simulink model "hiv_model_ekf"  (R2020b)
settings: Solver=VariableStepAuto  StartTime=0.0  StopTime=10.0  RelTol=1e-3
values from neighbouring files (symbols this model uses):
  Delta = 0.01    [init.m]
  P_0 = [diag((Theta*0.3).^2),zeros(6,3);zeros(3,9)]    [init.m]
  Theta = block.DialogPrm(2).Data    [hiv_model.m]    (also in init.m = [0.25 50 0.25 10 0.01 0.0045]')
  W_k = zeros(9,9)    [init.m]
  xdash0 = [1000 550 0.0001]'    [init.m]
  xdash12RL = block.DialogPrm(3).Data    [hiv_model.m]    (also in init.m = [1000 550]')
  Z_k = zeros(3,3);Z_k(1,1)=100;Z_k(2,2)=100;Z_k(3,3)=1e-5    [init.m]
undefined symbols (not defined in the file or in its folder): theta0
settings Model: Creator=schauer  LastModifiedBy=saleh

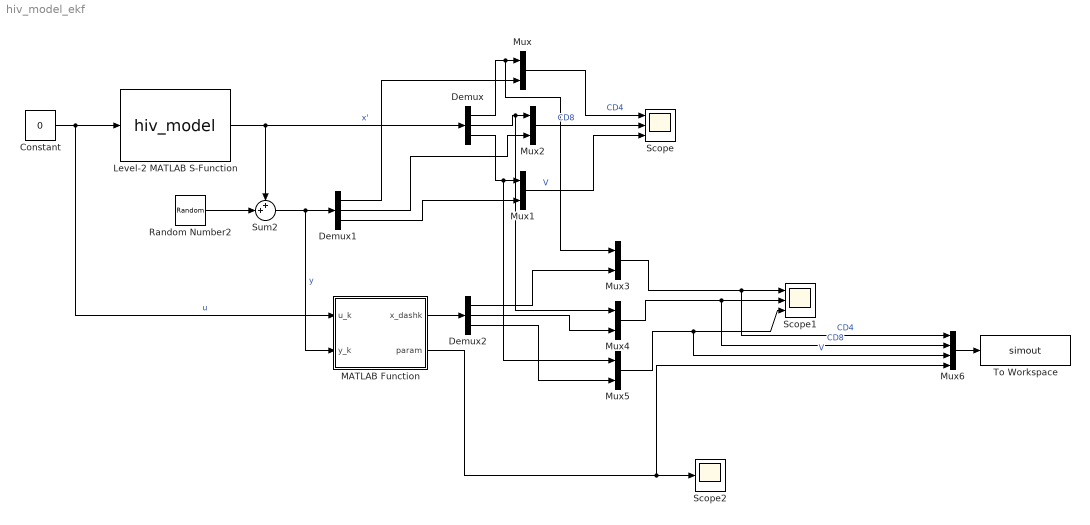
== system hiv_model_ekf ==
  Constant : Constant  Value=0
  Demux : Demux  Outputs=3
  Demux1 : Demux  Outputs=3
  Demux2 : Demux  Outputs=3
  Level-2 MATLAB S-Function : M-S-Function  FunctionName=hiv_model  Parameters=xdash0,Theta,xdash12RL
  MATLAB Function : MATLAB Function  TreatAsAtomicUnit=on  SystemSampleTime=Delta
  Mux{,1..5} (6 alike) : Mux  Inputs=2
  Mux6 : Mux
  Random Number2 : RandomNumber  Variance=[100 100 10^-5]  SampleTime=Delta
  Scope : Scope  NumInputPorts=3
  Scope1 : Scope  NumInputPorts=3
  Scope2 : Scope
  Sum2 : Sum  Inputs=++|
  To Workspace : ToWorkspace  VariableName=simout  SampleTime=-1
  wires:
  Constant/1 -> MATLAB Function/1(u_k), Level-2 MATLAB S-Function/1  "u"
  Level-2 MATLAB S-Function/1 -> Demux/1, Sum2/1  "x'"
  Mux/1 -> Scope/1  "CD4"
  Demux/1 -> Mux3/1, Mux/1
  Demux/3 -> Mux5/1, Mux1/1
  Mux1/1 -> Scope/3  "V"
  Sum2/1 -> MATLAB Function/2(y_k), Demux1/1  "y"
  Random Number2/1 -> Sum2/2
  Mux2/1 -> Scope/2  "CD8"
  Demux/2 -> Mux4/1, Mux2/1
  Demux1/1 -> Mux/2
  Demux1/2 -> Mux2/2
  Demux1/3 -> Mux1/2
  MATLAB Function/1(x_dashk) -> Demux2/1
  Demux2/1 -> Mux3/2
  Demux2/2 -> Mux4/2
  Demux2/3 -> Mux5/2
  Mux3/1 -> Mux6/1, Scope1/1  "CD4"
  Mux4/1 -> Mux6/2, Scope1/2  "CD8"
  Mux5/1 -> Mux6/3, Scope1/3  "V"
  MATLAB Function/2(param) -> Mux6/4, Scope2/1
  Mux6/1 -> To Workspace/1

== matlab function hiv_model_ekf/MATLAB Function ==
  settings: updateMethod=DISCRETE
  data: x_dashk output; param output; u_k input; y_k input; xdash0 parameter; P_0 parameter; W_k parameter; xdash12RL parameter; Delta parameter; Z_k parameter; theta0 parameter
function [x_dashk,param] = ekf(u_k,y_k,xdash0,P_0,W_k,xdash12RL,Delta,Z_k,theta0)
% Erweiterter Kalman Filter
% Zustände: x_dashk(x_k Strich/Ursprüngliche Zustände),6 Parameter
% 
 
 % Prädiktion initialisieren
 persistent x_k_p P_k_p 
 if isempty(x_k_p)
     x_k_p = ones(9,1);
     x_k_p(1:3,1) = xdash0;
     x_k_p(4:9,1) = theta0;
     P_k_p = P_0;
 end
 
 % Update
 % K berechnen
 C_k = [eye(3),zeros(3,6)];
 
 K_k = P_k_p*C_k'/(Z_k + C_k*P_k_p*C_k');
 x_k = x_k_p + K_k*(y_k-x_k_p(1:3));            % x_k_p(1:3) = h
 P_k = P_k_p - K_k*C_k*P_k_p + W_k;
 
 % Prädiktion updaten
 
 A_k = [(1-Delta*(x_k(4)-x_k(5)*x_k(3))),0,-Delta*x_k(4)*x_k(1),...
     Delta*(xdash12RL(1)-x_k(1)),Delta*x_k(1)*x_k(3),0,0,0,0;...                       % 1. Row
     0,(1-Delta*(x_k(6)+x_k(7)*x_k(3))),Delta*x_k(7)*x_k(2),0,0,...
     Delta*(xdash12RL(2)-x_k(2)),Delta*x_k(2)*x_k(3),0,0;...                           % 2. Row
     Delta*x_k(8)*x_k(3),-Delta*x_k(9)*x_k(3),1+Delta*(x_k(8)*x_k(1)-...
     x_k(9)*x_k(2)),0,0,0,0,Delta*x_k(1)*x_k(3),-Delta*x_k(2)*x_k(3);...    % 3. Row
     zeros(1,3),1,zeros(1,5);...                                            % 4. Row
     zeros(1,4),1,zeros(1,4);...                                            % 5. Row
     zeros(1,5),1,zeros(1,3);...                                            % 6. Row
     zeros(1,6),1,zeros(1,2);...                                            % 7. Row
     zeros(1,7),1,0;...                                                     % 8. Row
     zeros(1,8),1];
 
 x_kp1_p = [x_k(1)+Delta*(x_k(4)*(xdash12RL(1)-x_k(1))-x_k(5)*x_k(1)*x_k(3));...
     x_k(2)+Delta*(x_k(6)*(xdash12RL(2)-x_k(2))+x_k(7)*x_k(2)*x_k(3));...
     x_k(3)+Delta*(x_k(3)*(x_k(8)*x_k(1)-x_k(9)*x_k(2))-u_k);...
     x_k(4:9)];
 
 P_kp1_p = A_k*P_k*A_k' + W_k;
 
 x_k_p = x_kp1_p;
 P_k_p = P_kp1_p;
 
 x_dashk = x_k(1:3);
 param = x_k(4:9);
end
